simulink model "cst_robotarm"  (R2023b)
settings: Solver=ode23t  StartTime=0.0  StopTime=5  FixedStep=0.0001  MaxStep=0.05  RelTol=1e-3  EnableMultiTasking=on
model workspace (MAT data in the model file):
  DCMotor_J = 0.0946866703633
  DCMotor_K = 0.477771340295
  DCMotor_Kf = 0.921434142151
  DCMotor_L = 0.000316454712175
  DCMotor_R = 4.99938152603
  Ts = 0.1
  dFilt = [1 -0.1202]
  nFilt = [0.4399 0.4399]
undefined symbols (not defined in the file or in its folder): X, Y, Z
libraries: sm_lib x244, fl_lib x75, nesl_utility x28, ee_lib x21, slpidlib x6, SignalEditorBlockLib x1
(part 5 of 7)

== system cst_robotarm/6 DOF Robot Arm/6 DOF Robot Arm Mechanics/Hand/GripAttachmentPlate_1_RIGID ==
  ReferenceFrame : sm_lib/Frames and Transforms/Reference Frame
  Solid : sm_lib/Body Elements/File Solid  ExtGeomFileName=GripAttachmentPlate_Default_sldprt.STL  UnitType=Custom  ExtGeomFileUnits=mm  StepReaderType=HEX  ExportConvexHullGeometry=off  InertiaType=Custom  Mass=0.011413528336954156  MassUnits=kg  CenterOfMass=[0 0 1.5]  CenterOfMassUnits=mm  MomentsOfInertia=[0.70625654823604433 4.0114808704620435 4.7006171261926557]  MomentsOfInertiaUnits=kg*mm^2  ProductsOfInertia=[0 0 0]  ProductsOfInertiaUnits=kg*mm^2  BasedOnType=Density  Density=1000  DensityUnits=kg/(m^3)  DoExposeReferenceFrame=on  SerializedFrames=<Frames/>  GraphicType=FromGeometry  MarkerShape=Sphere  MarkerSize=10  MarkerSizeUnits=m  GraphicVisPropType=SimpleVisualProperties  GraphicDiffuseColor=[1.0 0.8 0.6]  GraphicSpecularColor=[0.5 0.5 0.5 1.0]  GraphicAmbientColor=[0.15 0.15 0.15 1.0]  GraphicEmissiveColor=[0.0 0.0 0.0 1.0]  GraphicShininess=75  GraphicOpacity=1
  F : PMIOPort  Side=Left
  connections:
  Solid/RConn1 -- ReferenceFrame/RConn1 -- F/RConn1

== system cst_robotarm/6 DOF Robot Arm/6 DOF Robot Arm Mechanics/Hand/ServoTJD2_1_RIGID ==
  ReferenceFrame : sm_lib/Frames and Transforms/Reference Frame
  Transform : sm_lib/Frames and Transforms/Rigid Transform  TranslationMethod=None  TranslationStandardOffset=0  TranslationStandardOffsetUnits=m  TranslationStandardAxis=+Z  TranslationCartesianOffset=[0 0 0]  TranslationCartesianOffsetUnits=m  TranslationROffset=0  TranslationROffsetUnits=m  TranslationZOffset=0  TranslationZOffsetUnits=m  TranslationThetaOffset=0  TranslationThetaOffsetUnits=deg  RotationMethod=None  RotationAngleUnits=deg  RotationStandardAxis=+Z  RotationAngle=0.0  RotationArbitraryAxis=[0 0 1]  FollAlignAxisA=+X  BaseAlignAxisA=+Y  FollAlignAxisB=+Y  BaseAlignAxisB=+Z  RotationSequenceAxes=FollowerAxes  RotationSequence=XYX  RotationSequenceAngles=[0 0 0]  RotationSequenceAnglesUnits=deg  RotationMatrix=[1 0 0; 0 1 0; 0 0 1]  Quaternion=[1 0 0 0]
  Transform1 : sm_lib/Frames and Transforms/Rigid Transform  TranslationMethod=Cartesian  TranslationStandardOffset=0  TranslationStandardOffsetUnits=mm  TranslationStandardAxis=+Z  TranslationCartesianOffset=[19.3675 9.8424999999999763 -1.1906249999999998]  TranslationCartesianOffsetUnits=mm  TranslationROffset=0  TranslationROffsetUnits=m  TranslationZOffset=0  TranslationZOffsetUnits=m  TranslationThetaOffset=0  TranslationThetaOffsetUnits=deg  RotationMethod=ArbitraryAxis  RotationAngleUnits=rad  RotationStandardAxis=+Z  RotationAngle=3.1415926535897931  RotationArbitraryAxis=[5.872382563893875e-17 -0.70710678118654746 -0.70710678118654757]  FollAlignAxisA=+X  BaseAlignAxisA=+Y  FollAlignAxisB=+Y  BaseAlignAxisB=+Z  RotationSequenceAxes=FollowerAxes  RotationSequence=XYX  RotationSequenceAngles=[0 0 0]  RotationSequenceAnglesUnits=deg  RotationMatrix=[1 0 0; 0 1 0; 0 0 1]  Quaternion=[1 0 0 0]
  Transform2 : sm_lib/Frames and Transforms/Rigid Transform  TranslationMethod=Cartesian  TranslationStandardOffset=0  TranslationStandardOffsetUnits=mm  TranslationStandardAxis=+Z  TranslationCartesianOffset=[19.367499999999982 9.8424999999999763 -23.8125]  TranslationCartesianOffsetUnits=mm  TranslationROffset=0  TranslationROffsetUnits=m  TranslationZOffset=0  TranslationZOffsetUnits=m  TranslationThetaOffset=0  TranslationThetaOffsetUnits=deg  RotationMethod=ArbitraryAxis  RotationAngleUnits=rad  RotationStandardAxis=+Z  RotationAngle=1.5707963267948968  RotationArbitraryAxis=[1 0 0]  FollAlignAxisA=+X  BaseAlignAxisA=+Y  FollAlignAxisB=+Y  BaseAlignAxisB=+Z  RotationSequenceAxes=FollowerAxes  RotationSequence=XYX  RotationSequenceAngles=[0 0 0]  RotationSequenceAnglesUnits=deg  RotationMatrix=[1 0 0; 0 1 0; 0 0 1]  Quaternion=[1 0 0 0]
  Transform3 : sm_lib/Frames and Transforms/Rigid Transform  TranslationMethod=Cartesian  TranslationStandardOffset=0  TranslationStandardOffsetUnits=mm  TranslationStandardAxis=+Z  TranslationCartesianOffset=[-8.9620000000000051 21.842499999999987 -9.8425000000000029]  TranslationCartesianOffsetUnits=mm  TranslationROffset=0  TranslationROffsetUnits=m  TranslationZOffset=0  TranslationZOffsetUnits=m  TranslationThetaOffset=0  TranslationThetaOffsetUnits=deg  RotationMethod=ArbitraryAxis  RotationAngleUnits=rad  RotationStandardAxis=+Z  RotationAngle=3.1415926535897931  RotationArbitraryAxis=[0.70710678118654746 -2.1920991699290503e-17 0.70710678118654757]  FollAlignAxisA=+X  BaseAlignAxisA=+Y  FollAlignAxisB=+Y  BaseAlignAxisB=+Z  RotationSequenceAxes=FollowerAxes  RotationSequence=XYX  RotationSequenceAngles=[0 0 0]  RotationSequenceAnglesUnits=deg  RotationMatrix=[1 0 0; 0 1 0; 0 0 1]  Quaternion=[1 0 0 0]
  bottom_cover_1_RIGID : Subsystem
  servo_Case_1_RIGID : Subsystem
  servo_cover_2_RIGID : Subsystem
  F : PMIOPort  Side=Right
  connections:
  Transform/RConn1 -- servo_cover_2_RIGID/LConn1
  Transform1/RConn1 -- servo_Case_1_RIGID/LConn1
  Transform2/RConn1 -- bottom_cover_1_RIGID/LConn1
  ReferenceFrame/RConn1 -- Transform/LConn1 -- Transform3/RConn1 -- Transform2/LConn1 -- Transform1/LConn1
  Transform3/LConn1 -- F/RConn1

== system cst_robotarm/6 DOF Robot Arm/6 DOF Robot Arm Mechanics/Hand/gat2_1_RIGID ==
  ReferenceFrame : sm_lib/Frames and Transforms/Reference Frame
  Solid : sm_lib/Body Elements/File Solid  ExtGeomFileName=gat2_Default_sldprt.STL  UnitType=Custom  ExtGeomFileUnits=mm  StepReaderType=HEX  ExportConvexHullGeometry=off  InertiaType=Custom  Mass=0.00050610242376002699  MassUnits=kg  CenterOfMass=[0 0 0]  CenterOfMassUnits=mm  MomentsOfInertia=[0.0015997718916707939 0.027019343024713809 0.028429326507474591]  MomentsOfInertiaUnits=kg*mm^2  ProductsOfInertia=[0 0 0]  ProductsOfInertiaUnits=kg*mm^2  BasedOnType=Density  Density=1000  DensityUnits=kg/(m^3)  DoExposeReferenceFrame=on  SerializedFrames=<Frames/>  GraphicType=FromGeometry  MarkerShape=Sphere  MarkerSize=10  MarkerSizeUnits=m  GraphicVisPropType=SimpleVisualProperties  GraphicDiffuseColor=[1.0 0.8 0.6]  GraphicSpecularColor=[0.5 0.5 0.5 1.0]  GraphicAmbientColor=[0.15 0.15 0.15 1.0]  GraphicEmissiveColor=[0.0 0.0 0.0 1.0]  GraphicShininess=75  GraphicOpacity=1
  F : PMIOPort  Side=Left
  connections:
  Solid/RConn1 -- ReferenceFrame/RConn1 -- F/RConn1

== system cst_robotarm/6 DOF Robot Arm/6 DOF Robot Arm Mechanics/Hand/gat2_2_RIGID ==
  ReferenceFrame : sm_lib/Frames and Transforms/Reference Frame
  Solid : sm_lib/Body Elements/File Solid  ExtGeomFileName=gat2_Default_sldprt.STL  UnitType=Custom  ExtGeomFileUnits=mm  StepReaderType=HEX  ExportConvexHullGeometry=off  InertiaType=Custom  Mass=0.00050610242376002699  MassUnits=kg  CenterOfMass=[0 0 0]  CenterOfMassUnits=mm  MomentsOfInertia=[0.0015997718916707939 0.027019343024713809 0.028429326507474591]  MomentsOfInertiaUnits=kg*mm^2  ProductsOfInertia=[0 0 0]  ProductsOfInertiaUnits=kg*mm^2  BasedOnType=Density  Density=1000  DensityUnits=kg/(m^3)  DoExposeReferenceFrame=on  SerializedFrames=<Frames/>  GraphicType=FromGeometry  MarkerShape=Sphere  MarkerSize=10  MarkerSizeUnits=m  GraphicVisPropType=SimpleVisualProperties  GraphicDiffuseColor=[1.0 0.8 0.6]  GraphicSpecularColor=[0.5 0.5 0.5 1.0]  GraphicAmbientColor=[0.15 0.15 0.15 1.0]  GraphicEmissiveColor=[0.0 0.0 0.0 1.0]  GraphicShininess=75  GraphicOpacity=1
  F : PMIOPort  Side=Left
  connections:
  Solid/RConn1 -- ReferenceFrame/RConn1 -- F/RConn1

== system cst_robotarm/6 DOF Robot Arm/6 DOF Robot Arm Mechanics/Hand/gat3_1_RIGID ==
  ReferenceFrame : sm_lib/Frames and Transforms/Reference Frame
  Solid : sm_lib/Body Elements/File Solid  ExtGeomFileName=gat3_Default_sldprt.STL  UnitType=Custom  ExtGeomFileUnits=mm  StepReaderType=HEX  ExportConvexHullGeometry=off  InertiaType=Custom  Mass=0.013404466225302725  MassUnits=kg  CenterOfMass=[2.3381498585899534 12.0054171558366 0]  CenterOfMassUnits=mm  MomentsOfInertia=[5.9325752245289687 5.0094665513353727 1.34350330449193]  MomentsOfInertiaUnits=kg*mm^2  ProductsOfInertia=[0 0 0.00016978260661059655]  ProductsOfInertiaUnits=kg*mm^2  BasedOnType=Density  Density=1000  DensityUnits=kg/(m^3)  DoExposeReferenceFrame=on  SerializedFrames=<Frames/>  GraphicType=FromGeometry  MarkerShape=Sphere  MarkerSize=10  MarkerSizeUnits=m  GraphicVisPropType=SimpleVisualProperties  GraphicDiffuseColor=[1.0 0.8 0.6]  GraphicSpecularColor=[0.5 0.5 0.5 1.0]  GraphicAmbientColor=[0.15 0.15 0.15 1.0]  GraphicEmissiveColor=[0.0 0.0 0.0 1.0]  GraphicShininess=75  GraphicOpacity=1
  F : PMIOPort  Side=Left
  connections:
  Solid/RConn1 -- ReferenceFrame/RConn1 -- F/RConn1

== system cst_robotarm/6 DOF Robot Arm/6 DOF Robot Arm Mechanics/Hand/lpags_02_1_RIGID ==
  ReferenceFrame : sm_lib/Frames and Transforms/Reference Frame
  SMLINK_HandGearXform : sm_lib/Frames and Transforms/Rigid Transform  TranslationMethod=None  TranslationStandardOffset=0  TranslationStandardOffsetUnits=m  TranslationStandardAxis=+Z  TranslationCartesianOffset=[0 0 0]  TranslationCartesianOffsetUnits=m  TranslationROffset=0  TranslationROffsetUnits=m  TranslationZOffset=0  TranslationZOffsetUnits=m  TranslationThetaOffset=0  TranslationThetaOffsetUnits=deg  RotationMethod=None  RotationAngleUnits=deg  RotationStandardAxis=+Z  RotationAngle=0.0  RotationArbitraryAxis=[0 0 1]  FollAlignAxisA=+X  BaseAlignAxisA=+Y  FollAlignAxisB=+Y  BaseAlignAxisB=+Z  RotationSequenceAxes=FollowerAxes  RotationSequence=XYX  RotationSequenceAngles=[0 0 0]  RotationSequenceAnglesUnits=deg  RotationMatrix=[1 0 0; 0 1 0; 0 0 1]  Quaternion=[1 0 0 0]
  Solid : sm_lib/Body Elements/File Solid  ExtGeomFileName=lpags-02_Default_sldprt.STL  UnitType=Custom  ExtGeomFileUnits=mm  StepReaderType=HEX  ExportConvexHullGeometry=off  InertiaType=Custom  Mass=0.0030318967834451023  MassUnits=kg  CenterOfMass=[0 0.57150000000000001 -0.00019934083817513303]  CenterOfMassUnits=mm  MomentsOfInertia=[0.31419992840808614 0.62773233420718355 0.31419225543277651]  MomentsOfInertiaUnits=kg*mm^2  ProductsOfInertia=[0 0 8.0061496389648527e-09]  ProductsOfInertiaUnits=kg*mm^2  BasedOnType=Density  Density=1000  DensityUnits=kg/(m^3)  DoExposeReferenceFrame=on  SerializedFrames=<Frames/>  GraphicType=FromGeometry  MarkerShape=Sphere  MarkerSize=10  MarkerSizeUnits=m  GraphicVisPropType=SimpleVisualProperties  GraphicDiffuseColor=[1.0 1.0 1.0]  GraphicSpecularColor=[0.5 0.5 0.5 1.0]  GraphicAmbientColor=[0.15 0.15 0.15 1.0]  GraphicEmissiveColor=[0.0 0.0 0.0 1.0]  GraphicShininess=75  GraphicOpacity=1
  F : PMIOPort  Side=Left
  SMLINK_HandGear : PMIOPort  Port=2  Side=Right
  connections:
  SMLINK_HandGearXform/LConn1 -- ReferenceFrame/RConn1 -- F/RConn1 -- Solid/RConn1
  SMLINK_HandGearXform/RConn1 -- SMLINK_HandGear/RConn1

== system cst_robotarm/6 DOF Robot Arm/6 DOF Robot Arm Mechanics/Turntable/ServoTJD_1_RIGID ==
  ReferenceFrame : sm_lib/Frames and Transforms/Reference Frame
  ServoHornPlastic_1_RIGID : Subsystem
  Transform : sm_lib/Frames and Transforms/Rigid Transform  TranslationMethod=None  TranslationStandardOffset=0  TranslationStandardOffsetUnits=m  TranslationStandardAxis=+Z  TranslationCartesianOffset=[0 0 0]  TranslationCartesianOffsetUnits=m  TranslationROffset=0  TranslationROffsetUnits=m  TranslationZOffset=0  TranslationZOffsetUnits=m  TranslationThetaOffset=0  TranslationThetaOffsetUnits=deg  RotationMethod=None  RotationAngleUnits=deg  RotationStandardAxis=+Z  RotationAngle=0.0  RotationArbitraryAxis=[0 0 1]  FollAlignAxisA=+X  BaseAlignAxisA=+Y  FollAlignAxisB=+Y  BaseAlignAxisB=+Z  RotationSequenceAxes=FollowerAxes  RotationSequence=XYX  RotationSequenceAngles=[0 0 0]  RotationSequenceAnglesUnits=deg  RotationMatrix=[1 0 0; 0 1 0; 0 0 1]  Quaternion=[1 0 0 0]
  Transform1 : sm_lib/Frames and Transforms/Rigid Transform  TranslationMethod=Cartesian  TranslationStandardOffset=0  TranslationStandardOffsetUnits=mm  TranslationStandardAxis=+Z  TranslationCartesianOffset=[19.367500000000003 9.8425000000000047 -1.1906250000000007]  TranslationCartesianOffsetUnits=mm  TranslationROffset=0  TranslationROffsetUnits=m  TranslationZOffset=0  TranslationZOffsetUnits=m  TranslationThetaOffset=0  TranslationThetaOffsetUnits=deg  RotationMethod=ArbitraryAxis  RotationAngleUnits=rad  RotationStandardAxis=+Z  RotationAngle=3.1415926535897931  RotationArbitraryAxis=[5.8878467200641572e-17 -0.70710678118654746 -0.70710678118654757]  FollAlignAxisA=+X  BaseAlignAxisA=+Y  FollAlignAxisB=+Y  BaseAlignAxisB=+Z  RotationSequenceAxes=FollowerAxes  RotationSequence=XYX  RotationSequenceAngles=[0 0 0]  RotationSequenceAnglesUnits=deg  RotationMatrix=[1 0 0; 0 1 0; 0 0 1]  Quaternion=[1 0 0 0]
  Transform2 : sm_lib/Frames and Transforms/Rigid Transform  TranslationMethod=Cartesian  TranslationStandardOffset=0  TranslationStandardOffsetUnits=mm  TranslationStandardAxis=+Z  TranslationCartesianOffset=[19.367499999999989 9.8425000000000047 -23.812500000000007]  TranslationCartesianOffsetUnits=mm  TranslationROffset=0  TranslationROffsetUnits=m  TranslationZOffset=0  TranslationZOffsetUnits=m  TranslationThetaOffset=0  TranslationThetaOffsetUnits=deg  RotationMethod=ArbitraryAxis  RotationAngleUnits=rad  RotationStandardAxis=+Z  RotationAngle=1.5707963267948968  RotationArbitraryAxis=[1 0 0]  FollAlignAxisA=+X  BaseAlignAxisA=+Y  FollAlignAxisB=+Y  BaseAlignAxisB=+Z  RotationSequenceAxes=FollowerAxes  RotationSequence=XYX  RotationSequenceAngles=[0 0 0]  RotationSequenceAnglesUnits=deg  RotationMatrix=[1 0 0; 0 1 0; 0 0 1]  Quaternion=[1 0 0 0]
  Transform3 : sm_lib/Frames and Transforms/Rigid Transform  TranslationMethod=Cartesian  TranslationStandardOffset=0  TranslationStandardOffsetUnits=mm  TranslationStandardAxis=+Z  TranslationCartesianOffset=[9.8425000000000029 9.8425000000000047 17.962]  TranslationCartesianOffsetUnits=mm  TranslationROffset=0  TranslationROffsetUnits=m  TranslationZOffset=0  TranslationZOffsetUnits=m  TranslationThetaOffset=0  TranslationThetaOffsetUnits=deg  RotationMethod=ArbitraryAxis  RotationAngleUnits=rad  RotationStandardAxis=+Z  RotationAngle=1.5707963267948968  RotationArbitraryAxis=[1 0 0]  FollAlignAxisA=+X  BaseAlignAxisA=+Y  FollAlignAxisB=+Y  BaseAlignAxisB=+Z  RotationSequenceAxes=FollowerAxes  RotationSequence=XYX  RotationSequenceAngles=[0 0 0]  RotationSequenceAnglesUnits=deg  RotationMatrix=[1 0 0; 0 1 0; 0 0 1]  Quaternion=[1 0 0 0]
  Transform4 : sm_lib/Frames and Transforms/Rigid Transform  TranslationMethod=Cartesian  TranslationStandardOffset=0  TranslationStandardOffsetUnits=mm  TranslationStandardAxis=+Z  TranslationCartesianOffset=[30.38750000000001 -48.386999999999396 8.9609000000000876]  TranslationCartesianOffsetUnits=mm  TranslationROffset=0  TranslationROffsetUnits=m  TranslationZOffset=0  TranslationZOffsetUnits=m  TranslationThetaOffset=0  TranslationThetaOffsetUnits=deg  RotationMethod=ArbitraryAxis  RotationAngleUnits=rad  RotationStandardAxis=+Z  RotationAngle=2.0943951023931939  RotationArbitraryAxis=[-0.5773502691896254 -0.57735026918962518 -0.57735026918962684]  FollAlignAxisA=+X  BaseAlignAxisA=+Y  FollAlignAxisB=+Y  BaseAlignAxisB=+Z  RotationSequenceAxes=FollowerAxes  RotationSequence=XYX  RotationSequenceAngles=[0 0 0]  RotationSequenceAnglesUnits=deg  RotationMatrix=[1 0 0; 0 1 0; 0 0 1]  Quaternion=[1 0 0 0]
  bottom_cover_1_RIGID : Subsystem
  servo_Case_1_RIGID : Subsystem
  servo_cover_2_RIGID : Subsystem
  F : PMIOPort  Side=Right
  connections:
  Transform/RConn1 -- servo_cover_2_RIGID/LConn1
  Transform1/RConn1 -- servo_Case_1_RIGID/LConn1
  Transform2/RConn1 -- bottom_cover_1_RIGID/LConn1
  ServoHornPlastic_1_RIGID/LConn1 -- Transform3/RConn1
  ReferenceFrame/RConn1 -- Transform/LConn1 -- Transform1/LConn1 -- Transform4/RConn1 -- Transform3/LConn1 -- Transform2/LConn1
  Transform4/LConn1 -- F/RConn1

== system cst_robotarm/6 DOF Robot Arm/6 DOF Robot Arm Mechanics/Turntable/ServoTJD_2_RIGID ==
  ReferenceFrame : sm_lib/Frames and Transforms/Reference Frame
  ServoHornPlastic_1_RIGID : Subsystem
  Transform : sm_lib/Frames and Transforms/Rigid Transform  TranslationMethod=None  TranslationStandardOffset=0  TranslationStandardOffsetUnits=m  TranslationStandardAxis=+Z  TranslationCartesianOffset=[0 0 0]  TranslationCartesianOffsetUnits=m  TranslationROffset=0  TranslationROffsetUnits=m  TranslationZOffset=0  TranslationZOffsetUnits=m  TranslationThetaOffset=0  TranslationThetaOffsetUnits=deg  RotationMethod=None  RotationAngleUnits=deg  RotationStandardAxis=+Z  RotationAngle=0.0  RotationArbitraryAxis=[0 0 1]  FollAlignAxisA=+X  BaseAlignAxisA=+Y  FollAlignAxisB=+Y  BaseAlignAxisB=+Z  RotationSequenceAxes=FollowerAxes  RotationSequence=XYX  RotationSequenceAngles=[0 0 0]  RotationSequenceAnglesUnits=deg  RotationMatrix=[1 0 0; 0 1 0; 0 0 1]  Quaternion=[1 0 0 0]
  Transform1 : sm_lib/Frames and Transforms/Rigid Transform  TranslationMethod=Cartesian  TranslationStandardOffset=0  TranslationStandardOffsetUnits=mm  TranslationStandardAxis=+Z  TranslationCartesianOffset=[19.36750000000001 9.8424999999999905 -1.1906250000000007]  TranslationCartesianOffsetUnits=mm  TranslationROffset=0  TranslationROffsetUnits=m  TranslationZOffset=0  TranslationZOffsetUnits=m  TranslationThetaOffset=0  TranslationThetaOffsetUnits=deg  RotationMethod=ArbitraryAxis  RotationAngleUnits=rad  RotationStandardAxis=+Z  RotationAngle=3.1415926535897931  RotationArbitraryAxis=[4.5974986977188573e-17 -0.70710678118654746 -0.70710678118654757]  FollAlignAxisA=+X  BaseAlignAxisA=+Y  FollAlignAxisB=+Y  BaseAlignAxisB=+Z  RotationSequenceAxes=FollowerAxes  RotationSequence=XYX  RotationSequenceAngles=[0 0 0]  RotationSequenceAnglesUnits=deg  RotationMatrix=[1 0 0; 0 1 0; 0 0 1]  Quaternion=[1 0 0 0]
  Transform2 : sm_lib/Frames and Transforms/Rigid Transform  TranslationMethod=Cartesian  TranslationStandardOffset=0  TranslationStandardOffsetUnits=mm  TranslationStandardAxis=+Z  TranslationCartesianOffset=[19.367499999999993 9.8425000000000047 -23.8125]  TranslationCartesianOffsetUnits=mm  TranslationROffset=0  TranslationROffsetUnits=m  TranslationZOffset=0  TranslationZOffsetUnits=m  TranslationThetaOffset=0  TranslationThetaOffsetUnits=deg  RotationMethod=ArbitraryAxis  RotationAngleUnits=rad  RotationStandardAxis=+Z  RotationAngle=1.5707963267948968  RotationArbitraryAxis=[1 0 0]  FollAlignAxisA=+X  BaseAlignAxisA=+Y  FollAlignAxisB=+Y  BaseAlignAxisB=+Z  RotationSequenceAxes=FollowerAxes  RotationSequence=XYX  RotationSequenceAngles=[0 0 0]  RotationSequenceAnglesUnits=deg  RotationMatrix=[1 0 0; 0 1 0; 0 0 1]  Quaternion=[1 0 0 0]
  Transform3 : sm_lib/Frames and Transforms/Rigid Transform  TranslationMethod=Cartesian  TranslationStandardOffset=0  TranslationStandardOffsetUnits=mm  TranslationStandardAxis=+Z  TranslationCartesianOffset=[9.8425000000000047 9.8424999999999905 17.962000000000007]  TranslationCartesianOffsetUnits=mm  TranslationROffset=0  TranslationROffsetUnits=m  TranslationZOffset=0  TranslationZOffsetUnits=m  TranslationThetaOffset=0  TranslationThetaOffsetUnits=deg  RotationMethod=ArbitraryAxis  RotationAngleUnits=rad  RotationStandardAxis=+Z  RotationAngle=1.5707963267948968  RotationArbitraryAxis=[1 0 0]  FollAlignAxisA=+X  BaseAlignAxisA=+Y  FollAlignAxisB=+Y  BaseAlignAxisB=+Z  RotationSequenceAxes=FollowerAxes  RotationSequence=XYX  RotationSequenceAngles=[0 0 0]  RotationSequenceAnglesUnits=deg  RotationMatrix=[1 0 0; 0 1 0; 0 0 1]  Quaternion=[1 0 0 0]
  Transform4 : sm_lib/Frames and Transforms/Rigid Transform  TranslationMethod=Cartesian  TranslationStandardOffset=0  TranslationStandardOffsetUnits=mm  TranslationStandardAxis=+Z  TranslationCartesianOffset=[30.387499999999971 2.4257000000008517 8.9608999999998762]  TranslationCartesianOffsetUnits=mm  TranslationROffset=0  TranslationROffsetUnits=m  TranslationZOffset=0  TranslationZOffsetUnits=m  TranslationThetaOffset=0  TranslationThetaOffsetUnits=deg  RotationMethod=ArbitraryAxis  RotationAngleUnits=rad  RotationStandardAxis=+Z  RotationAngle=2.0943951023931944  RotationArbitraryAxis=[-0.57735026918962506 -0.57735026918962529 -0.57735026918962684]  FollAlignAxisA=+X  BaseAlignAxisA=+Y  FollAlignAxisB=+Y  BaseAlignAxisB=+Z  RotationSequenceAxes=FollowerAxes  RotationSequence=XYX  RotationSequenceAngles=[0 0 0]  RotationSequenceAnglesUnits=deg  RotationMatrix=[1 0 0; 0 1 0; 0 0 1]  Quaternion=[1 0 0 0]
  bottom_cover_1_RIGID : Subsystem
  servo_Case_1_RIGID : Subsystem
  servo_cover_2_RIGID : Subsystem
  F : PMIOPort  Side=Right
  connections:
  Transform/RConn1 -- servo_cover_2_RIGID/LConn1
  Transform1/RConn1 -- servo_Case_1_RIGID/LConn1
  Transform2/RConn1 -- bottom_cover_1_RIGID/LConn1
  ServoHornPlastic_1_RIGID/LConn1 -- Transform3/RConn1
  Transform/LConn1 -- ReferenceFrame/RConn1 -- Transform4/RConn1 -- Transform3/LConn1 -- Transform2/LConn1 -- Transform1/LConn1
  Transform4/LConn1 -- F/RConn1

== system cst_robotarm/6 DOF Robot Arm/6 DOF Robot Arm Mechanics/Turntable/TurntableBase_1_RIGID ==
  ReferenceFrame : sm_lib/Frames and Transforms/Reference Frame
  Solid : sm_lib/Body Elements/File Solid  ExtGeomFileName=TurntableBase_Default_sldprt.STL  UnitType=Custom  ExtGeomFileUnits=mm  StepReaderType=HEX  ExportConvexHullGeometry=off  InertiaType=Custom  Mass=0.061984090111562314  MassUnits=kg  CenterOfMass=[0 8.3537655787743348e-13 -9.8678648861571805]  CenterOfMassUnits=mm  MomentsOfInertia=[22.766528568089555 51.610594449827772 34.871884065003805]  MomentsOfInertiaUnits=kg*mm^2  ProductsOfInertia=[0 0 0]  ProductsOfInertiaUnits=kg*mm^2  BasedOnType=Density  Density=1000  DensityUnits=kg/(m^3)  DoExposeReferenceFrame=on  SerializedFrames=<Frames/>  GraphicType=FromGeometry  MarkerShape=Sphere  MarkerSize=10  MarkerSizeUnits=m  GraphicVisPropType=SimpleVisualProperties  GraphicDiffuseColor=[0.8 0.8 0.8]  GraphicSpecularColor=[0.5 0.5 0.5 1.0]  GraphicAmbientColor=[0.15 0.15 0.15 1.0]  GraphicEmissiveColor=[0.0 0.0 0.0 1.0]  GraphicShininess=75  GraphicOpacity=1
  F : PMIOPort  Side=Left
  connections:
  Solid/RConn1 -- ReferenceFrame/RConn1 -- F/RConn1

== system cst_robotarm/6 DOF Robot Arm/6 DOF Robot Arm Mechanics/Turntable/TurntablePlate_1_RIGID ==
  ReferenceFrame : sm_lib/Frames and Transforms/Reference Frame
  Solid : sm_lib/Body Elements/File Solid  ExtGeomFileName=TurntablePlate_Default_sldprt.STL  UnitType=Custom  ExtGeomFileUnits=mm  StepReaderType=HEX  ExportConvexHullGeometry=off  InertiaType=Custom  Mass=0.017394579990693507  MassUnits=kg  CenterOfMass=[28.782349121413723 2.6365798461097167 -30.489563019987546]  CenterOfMassUnits=mm  MomentsOfInertia=[6.1456876544929333 11.14133340240272 5.8740116461995679]  MomentsOfInertiaUnits=kg*mm^2  ProductsOfInertia=[-0.010484087253259841 -0.065628305606111978 0.0066466281662198451]  ProductsOfInertiaUnits=kg*mm^2  BasedOnType=Density  Density=1000  DensityUnits=kg/(m^3)  DoExposeReferenceFrame=on  SerializedFrames=<Frames/>  GraphicType=FromGeometry  MarkerShape=Sphere  MarkerSize=10  MarkerSizeUnits=m  GraphicVisPropType=SimpleVisualProperties  GraphicDiffuseColor=[0.8 0.8 0.8]  GraphicSpecularColor=[0.5 0.5 0.5 1.0]  GraphicAmbientColor=[0.15 0.15 0.15 1.0]  GraphicEmissiveColor=[0.0 0.0 0.0 1.0]  GraphicShininess=75  GraphicOpacity=1
  F : PMIOPort  Side=Left
  connections:
  Solid/RConn1 -- ReferenceFrame/RConn1 -- F/RConn1

== system cst_robotarm/6 DOF Robot Arm/6 DOF Robot Arm Mechanics/Wrist/MotorWristAsm_1_RIGID ==
  BB_01_1_RIGID : Subsystem
  ReferenceFrame : sm_lib/Frames and Transforms/Reference Frame
  ServoTJD2_1_RIGID : Subsystem
  Transform : sm_lib/Frames and Transforms/Rigid Transform  TranslationMethod=Cartesian  TranslationStandardOffset=0  TranslationStandardOffsetUnits=mm  TranslationStandardAxis=+Z  TranslationCartesianOffset=[49.387968408803829 0 4.318000000000044]  TranslationCartesianOffsetUnits=mm  TranslationROffset=0  TranslationROffsetUnits=m  TranslationZOffset=0  TranslationZOffsetUnits=m  TranslationThetaOffset=0  TranslationThetaOffsetUnits=deg  RotationMethod=ArbitraryAxis  RotationAngleUnits=rad  RotationStandardAxis=+Z  RotationAngle=2.0943951023931953  RotationArbitraryAxis=[0.57735026918962573 0.57735026918962573 0.57735026918962584]  FollAlignAxisA=+X  BaseAlignAxisA=+Y  FollAlignAxisB=+Y  BaseAlignAxisB=+Z  RotationSequenceAxes=FollowerAxes  RotationSequence=XYX  RotationSequenceAngles=[0 0 0]  RotationSequenceAnglesUnits=deg  RotationMatrix=[1 0 0; 0 1 0; 0 0 1]  Quaternion=[1 0 0 0]
  Transform1 : sm_lib/Frames and Transforms/Rigid Transform  TranslationMethod=Cartesian  TranslationStandardOffset=0  TranslationStandardOffsetUnits=mm  TranslationStandardAxis=+Z  TranslationCartesianOffset=[8.9130684088038343 49.720500000000008 5.8420000000000138]  TranslationCartesianOffsetUnits=mm  TranslationROffset=0  TranslationROffsetUnits=m  TranslationZOffset=0  TranslationZOffsetUnits=m  TranslationThetaOffset=0  TranslationThetaOffsetUnits=deg  RotationMethod=None  RotationAngleUnits=deg  RotationStandardAxis=+Z  RotationAngle=0.0  RotationArbitraryAxis=[0 0 1]  FollAlignAxisA=+X  BaseAlignAxisA=+Y  FollAlignAxisB=+Y  BaseAlignAxisB=+Z  RotationSequenceAxes=FollowerAxes  RotationSequence=XYX  RotationSequenceAngles=[0 0 0]  RotationSequenceAnglesUnits=deg  RotationMatrix=[1 0 0; 0 1 0; 0 0 1]  Quaternion=[1 0 0 0]
  Transform2 : sm_lib/Frames and Transforms/Rigid Transform  TranslationMethod=Cartesian  TranslationStandardOffset=0  TranslationStandardOffsetUnits=mm  TranslationStandardAxis=+Z  TranslationCartesianOffset=[-49.720500000000015 4.318000000000044 8.913068408803829]  TranslationCartesianOffsetUnits=mm  TranslationROffset=0  TranslationROffsetUnits=m  TranslationZOffset=0  TranslationZOffsetUnits=m  TranslationThetaOffset=0  TranslationThetaOffsetUnits=deg  RotationMethod=ArbitraryAxis  RotationAngleUnits=rad  RotationStandardAxis=+Z  RotationAngle=2.0943951023931953  RotationArbitraryAxis=[0.57735026918962584 0.57735026918962573 -0.57735026918962573]  FollAlignAxisA=+X  BaseAlignAxisA=+Y  FollAlignAxisB=+Y  BaseAlignAxisB=+Z  RotationSequenceAxes=FollowerAxes  RotationSequence=XYX  RotationSequenceAngles=[0 0 0]  RotationSequenceAnglesUnits=deg  RotationMatrix=[1 0 0; 0 1 0; 0 0 1]  Quaternion=[1 0 0 0]
  asb_14_2_RIGID : Subsystem
  F : PMIOPort  Side=Right
  connections:
  Transform/RConn1 -- asb_14_2_RIGID/LConn1
  BB_01_1_RIGID/LConn1 -- Transform1/RConn1
  ReferenceFrame/RConn1 -- ServoTJD2_1_RIGID/LConn1 -- Transform2/RConn1 -- Transform1/LConn1 -- Transform/LConn1
  Transform2/LConn1 -- F/RConn1

== system cst_robotarm/6 DOF Robot Arm/6 DOF Robot Arm Mechanics/Wrist/asb_09_1_RIGID ==
  ReferenceFrame : sm_lib/Frames and Transforms/Reference Frame
  Solid : sm_lib/Body Elements/File Solid  ExtGeomFileName=asb-09_Default_sldprt.STL  UnitType=Custom  ExtGeomFileUnits=mm  StepReaderType=HEX  ExportConvexHullGeometry=off  InertiaType=Custom  Mass=0.012849741350911532  MassUnits=kg  CenterOfMass=[0 11.553213185970444 0]  CenterOfMassUnits=mm  MomentsOfInertia=[2.609817980818478 6.7181730593401783 8.0141886683045769]  MomentsOfInertiaUnits=kg*mm^2  ProductsOfInertia=[0 0 0]  ProductsOfInertiaUnits=kg*mm^2  BasedOnType=Density  Density=1000  DensityUnits=kg/(m^3)  DoExposeReferenceFrame=on  SerializedFrames=<Frames/>  GraphicType=FromGeometry  MarkerShape=Sphere  MarkerSize=10  MarkerSizeUnits=m  GraphicVisPropType=SimpleVisualProperties  GraphicDiffuseColor=[0.8 1.0 0.6]  GraphicSpecularColor=[0.5 0.5 0.5 1.0]  GraphicAmbientColor=[0.15 0.15 0.15 1.0]  GraphicEmissiveColor=[0.0 0.0 0.0 1.0]  GraphicShininess=75  GraphicOpacity=1
  F : PMIOPort  Side=Left
  connections:
  Solid/RConn1 -- ReferenceFrame/RConn1 -- F/RConn1

== system cst_robotarm/6 DOF Robot Arm/DC Motors/Bicep Motor1/Power Amplifier ==
  Duty : Inport
  REV : Inport  Port=2
  BRK : Inport  Port=3
  Controlled PWM Voltage : ee_lib/Integrated Circuits/Controlled PWM Voltage  F=400 Hz  TD=0 s  pulse_width_offset=0 s  pulse_min=0 s  pwm_or_av=2  event_type=1  sample_time=1e-6 s  Vmin=0 V  Vmax=5 V  Vm=5 V  u_min=0  u_max=1
  Electrical Reference1 : fl_lib/Electrical/Electrical Elements/Electrical Reference
  H-Bridge : ee_lib/Semiconductors & Converters/Converters/H-Bridge  supply_ports=ee.enum.supply_ports.hidesupply  pwm_or_av=2  regenerative_braking_mode=2  discontinuous=0  freewheeling_mode=1  Rload=10 Ohm  Lload=1e-5 H  F=10 kHz  Venable=2.5 V  Vmax=5 V  Vreverse=2.5 V  Vbrake=2.5 V  Vm=12 V  Ron=0.1 Ohm  Don=0.05 Ohm  Goff=1e-6 S  Tmeas=298.15 K  Ron2=0.1 Ohm  Don2=0.05 Ohm  Tmeas2=398.15 K  thermal_mass=100 J/K  initial_temperature=298.15 K
  SL2Vbrk : Subsystem
  SL2Vduty : Subsystem
  SL2Vrev : Subsystem
  V + : PMIOPort  Tag=PMCPort  Side=Right
  V -- : PMIOPort  Tag=PMCPort  Port=2  Side=Right
  wires:
  BRK/1 -> SL2Vbrk/1(Signal)
  REV/1 -> SL2Vrev/1(Signal)
  Duty/1 -> SL2Vduty/1(Signal)
  connections:
  SL2Vbrk/RConn1 -- H-Bridge/LConn4
  H-Bridge/LConn1 -- Controlled PWM Voltage/RConn1
  SL2Vduty/RConn1 -- Controlled PWM Voltage/LConn1
  H-Bridge/RConn1 -- V +/RConn1
  SL2Vrev/RConn1 -- H-Bridge/LConn3
  H-Bridge/LConn2 -- Controlled PWM Voltage/LConn2 -- Electrical Reference1/LConn1 -- V --/RConn1 -- H-Bridge/RConn2 -- Controlled PWM Voltage/RConn2

== system cst_robotarm/6 DOF Robot Arm/DC Motors/Bicep Motor2/Power Amplifier ==
  Duty : Inport
  REV : Inport  Port=2
  BRK : Inport  Port=3
  Controlled PWM Voltage : ee_lib/Integrated Circuits/Controlled PWM Voltage  F=400 Hz  TD=0 s  pulse_width_offset=0 s  pulse_min=0 s  pwm_or_av=2  event_type=1  sample_time=1e-6 s  Vmin=0 V  Vmax=5 V  Vm=5 V  u_min=0  u_max=1
  Electrical Reference1 : fl_lib/Electrical/Electrical Elements/Electrical Reference
  H-Bridge : ee_lib/Semiconductors & Converters/Converters/H-Bridge  supply_ports=ee.enum.supply_ports.hidesupply  pwm_or_av=2  regenerative_braking_mode=2  discontinuous=0  freewheeling_mode=1  Rload=10 Ohm  Lload=1e-5 H  F=10 kHz  Venable=2.5 V  Vmax=5 V  Vreverse=2.5 V  Vbrake=2.5 V  Vm=12 V  Ron=0.1 Ohm  Don=0.05 Ohm  Goff=1e-6 S  Tmeas=298.15 K  Ron2=0.1 Ohm  Don2=0.05 Ohm  Tmeas2=398.15 K  thermal_mass=100 J/K  initial_temperature=298.15 K
  SL2Vbrk : Subsystem
  SL2Vduty : Subsystem
  SL2Vrev : Subsystem
  V + : PMIOPort  Tag=PMCPort  Side=Right
  V -- : PMIOPort  Tag=PMCPort  Port=2  Side=Right
  wires:
  Duty/1 -> SL2Vduty/1(Signal)
  REV/1 -> SL2Vrev/1(Signal)
  BRK/1 -> SL2Vbrk/1(Signal)
  connections:
  Controlled PWM Voltage/RConn2 -- H-Bridge/RConn2 -- V --/RConn1 -- Electrical Reference1/LConn1 -- Controlled PWM Voltage/LConn2 -- H-Bridge/LConn2
  SL2Vrev/RConn1 -- H-Bridge/LConn3
  H-Bridge/RConn1 -- V +/RConn1
  SL2Vduty/RConn1 -- Controlled PWM Voltage/LConn1
  H-Bridge/LConn1 -- Controlled PWM Voltage/RConn1
  SL2Vbrk/RConn1 -- H-Bridge/LConn4

== system cst_robotarm/6 DOF Robot Arm/DC Motors/Forearm Motor/Power Amplifier ==
  Duty : Inport
  REV : Inport  Port=2
  BRK : Inport  Port=3
  Controlled PWM Voltage : ee_lib/Integrated Circuits/Controlled PWM Voltage  F=400 Hz  TD=0 s  pulse_width_offset=0 s  pulse_min=0 s  pwm_or_av=2  event_type=1  sample_time=1e-6 s  Vmin=0 V  Vmax=5 V  Vm=5 V  u_min=0  u_max=1
  Electrical Reference1 : fl_lib/Electrical/Electrical Elements/Electrical Reference
  H-Bridge : ee_lib/Semiconductors & Converters/Converters/H-Bridge  supply_ports=ee.enum.supply_ports.hidesupply  pwm_or_av=2  regenerative_braking_mode=2  discontinuous=0  freewheeling_mode=1  Rload=10 Ohm  Lload=1e-5 H  F=10 kHz  Venable=2.5 V  Vmax=5 V  Vreverse=2.5 V  Vbrake=2.5 V  Vm=12 V  Ron=0.1 Ohm  Don=0.05 Ohm  Goff=1e-6 S  Tmeas=298.15 K  Ron2=0.1 Ohm  Don2=0.05 Ohm  Tmeas2=398.15 K  thermal_mass=100 J/K  initial_temperature=298.15 K
  SL2Vbrk : Subsystem
  SL2Vduty : Subsystem
  SL2Vrev : Subsystem
  V + : PMIOPort  Tag=PMCPort  Side=Right
  V -- : PMIOPort  Tag=PMCPort  Port=2  Side=Right
  wires:
  Duty/1 -> SL2Vduty/1(Signal)
  REV/1 -> SL2Vrev/1(Signal)
  BRK/1 -> SL2Vbrk/1(Signal)
  connections:
  Controlled PWM Voltage/RConn2 -- H-Bridge/RConn2 -- V --/RConn1 -- Electrical Reference1/LConn1 -- Controlled PWM Voltage/LConn2 -- H-Bridge/LConn2
  SL2Vrev/RConn1 -- H-Bridge/LConn3
  H-Bridge/RConn1 -- V +/RConn1
  SL2Vduty/RConn1 -- Controlled PWM Voltage/LConn1
  H-Bridge/LConn1 -- Controlled PWM Voltage/RConn1
  SL2Vbrk/RConn1 -- H-Bridge/LConn4

== system cst_robotarm/6 DOF Robot Arm/DC Motors/Hand Motor/Power Amplifier ==
  Duty : Inport
  REV : Inport  Port=2
  BRK : Inport  Port=3
  Controlled PWM Voltage : ee_lib/Integrated Circuits/Controlled PWM Voltage  F=400 Hz  TD=0 s  pulse_width_offset=0 s  pulse_min=0 s  pwm_or_av=2  event_type=1  sample_time=1e-6 s  Vmin=0 V  Vmax=5 V  Vm=5 V  u_min=0  u_max=1
  Electrical Reference1 : fl_lib/Electrical/Electrical Elements/Electrical Reference
  H-Bridge : ee_lib/Semiconductors & Converters/Converters/H-Bridge  supply_ports=ee.enum.supply_ports.hidesupply  pwm_or_av=2  regenerative_braking_mode=2  discontinuous=0  freewheeling_mode=1  Rload=10 Ohm  Lload=1e-5 H  F=10 kHz  Venable=2.5 V  Vmax=5 V  Vreverse=2.5 V  Vbrake=2.5 V  Vm=12 V  Ron=0.1 Ohm  Don=0.05 Ohm  Goff=1e-6 S  Tmeas=298.15 K  Ron2=0.1 Ohm  Don2=0.05 Ohm  Tmeas2=398.15 K  thermal_mass=100 J/K  initial_temperature=298.15 K
  SL2Vbrk : Subsystem
  SL2Vduty : Subsystem
  SL2Vrev : Subsystem
  V + : PMIOPort  Tag=PMCPort  Side=Right
  V -- : PMIOPort  Tag=PMCPort  Port=2  Side=Right
  wires:
  Duty/1 -> SL2Vduty/1(Signal)
  REV/1 -> SL2Vrev/1(Signal)
  BRK/1 -> SL2Vbrk/1(Signal)
  connections:
  Controlled PWM Voltage/RConn2 -- H-Bridge/RConn2 -- V --/RConn1 -- Electrical Reference1/LConn1 -- Controlled PWM Voltage/LConn2 -- H-Bridge/LConn2
  SL2Vrev/RConn1 -- H-Bridge/LConn3
  H-Bridge/RConn1 -- V +/RConn1
  SL2Vduty/RConn1 -- Controlled PWM Voltage/LConn1
  H-Bridge/LConn1 -- Controlled PWM Voltage/RConn1
  SL2Vbrk/RConn1 -- H-Bridge/LConn4

== system cst_robotarm/6 DOF Robot Arm/DC Motors/Hand Motor1/Power Amplifier ==
  Duty : Inport
  REV : Inport  Port=2
  BRK : Inport  Port=3
  Controlled PWM Voltage : ee_lib/Integrated Circuits/Controlled PWM Voltage  F=400 Hz  TD=0 s  pulse_width_offset=0 s  pulse_min=0 s  pwm_or_av=2  event_type=1  sample_time=1e-6 s  Vmin=0 V  Vmax=5 V  Vm=5 V  u_min=0  u_max=1
  Electrical Reference1 : fl_lib/Electrical/Electrical Elements/Electrical Reference
  H-Bridge : ee_lib/Semiconductors & Converters/Converters/H-Bridge  supply_ports=ee.enum.supply_ports.hidesupply  pwm_or_av=2  regenerative_braking_mode=2  discontinuous=0  freewheeling_mode=1  Rload=10 Ohm  Lload=1e-5 H  F=10 kHz  Venable=2.5 V  Vmax=5 V  Vreverse=2.5 V  Vbrake=2.5 V  Vm=12 V  Ron=0.1 Ohm  Don=0.05 Ohm  Goff=1e-6 S  Tmeas=298.15 K  Ron2=0.1 Ohm  Don2=0.05 Ohm  Tmeas2=398.15 K  thermal_mass=100 J/K  initial_temperature=298.15 K
  SL2Vbrk : Subsystem
  SL2Vduty : Subsystem
  SL2Vrev : Subsystem
  V + : PMIOPort  Tag=PMCPort  Side=Right
  V -- : PMIOPort  Tag=PMCPort  Port=2  Side=Right
  wires:
  BRK/1 -> SL2Vbrk/1(Signal)
  REV/1 -> SL2Vrev/1(Signal)
  Duty/1 -> SL2Vduty/1(Signal)
  connections:
  SL2Vbrk/RConn1 -- H-Bridge/LConn4
  H-Bridge/LConn1 -- Controlled PWM Voltage/RConn1
  SL2Vduty/RConn1 -- Controlled PWM Voltage/LConn1
  H-Bridge/RConn1 -- V +/RConn1
  SL2Vrev/RConn1 -- H-Bridge/LConn3
  H-Bridge/LConn2 -- Controlled PWM Voltage/LConn2 -- Electrical Reference1/LConn1 -- V --/RConn1 -- H-Bridge/RConn2 -- Controlled PWM Voltage/RConn2

== system cst_robotarm/6 DOF Robot Arm/DC Motors/Turntable Motor/Power Amplifier ==
  Duty : Inport
  REV : Inport  Port=2
  BRK : Inport  Port=3
  Controlled PWM Voltage : ee_lib/Integrated Circuits/Controlled PWM Voltage  F=400 Hz  TD=0 s  pulse_width_offset=0 s  pulse_min=0 s  pwm_or_av=2  event_type=1  sample_time=1e-6 s  Vmin=0 V  Vmax=5 V  Vm=5 V  u_min=0  u_max=1
  Electrical Reference1 : fl_lib/Electrical/Electrical Elements/Electrical Reference
  H-Bridge : ee_lib/Semiconductors & Converters/Converters/H-Bridge  supply_ports=ee.enum.supply_ports.hidesupply  pwm_or_av=2  regenerative_braking_mode=2  discontinuous=0  freewheeling_mode=1  Rload=10 Ohm  Lload=1e-5 H  F=10 kHz  Venable=2.5 V  Vmax=5 V  Vreverse=2.5 V  Vbrake=2.5 V  Vm=12 V  Ron=0.1 Ohm  Don=0.05 Ohm  Goff=1e-6 S  Tmeas=298.15 K  Ron2=0.1 Ohm  Don2=0.05 Ohm  Tmeas2=398.15 K  thermal_mass=100 J/K  initial_temperature=298.15 K
  SL2Vbrk : Subsystem
  SL2Vduty : Subsystem
  SL2Vrev : Subsystem
  Scope : Scope  NumInputPorts=4
  V + : PMIOPort  Tag=PMCPort  Side=Right
  V -- : PMIOPort  Tag=PMCPort  Port=2  Side=Right
  wires:
  Duty/1 -> Scope/3, SL2Vduty/1(Signal)
  REV/1 -> Scope/2, SL2Vrev/1(Signal)
  BRK/1 -> Scope/4, SL2Vbrk/1(Signal)
  connections:
  Controlled PWM Voltage/RConn2 -- H-Bridge/RConn2 -- V --/RConn1 -- Electrical Reference1/LConn1 -- Controlled PWM Voltage/LConn2 -- H-Bridge/LConn2
  SL2Vrev/RConn1 -- H-Bridge/LConn3
  H-Bridge/RConn1 -- V +/RConn1
  SL2Vduty/RConn1 -- Controlled PWM Voltage/LConn1
  H-Bridge/LConn1 -- Controlled PWM Voltage/RConn1
  SL2Vbrk/RConn1 -- H-Bridge/LConn4

== system cst_robotarm/6 DOF Robot Arm/DC Motors/Wrist Motor/Power Amplifier ==
  Duty : Inport
  REV : Inport  Port=2
  BRK : Inport  Port=3
  Controlled PWM Voltage : ee_lib/Integrated Circuits/Controlled PWM Voltage  F=400 Hz  TD=0 s  pulse_width_offset=0 s  pulse_min=0 s  pwm_or_av=2  event_type=1  sample_time=1e-6 s  Vmin=0 V  Vmax=5 V  Vm=5 V  u_min=0  u_max=1
  Electrical Reference1 : fl_lib/Electrical/Electrical Elements/Electrical Reference
  H-Bridge : ee_lib/Semiconductors & Converters/Converters/H-Bridge  supply_ports=ee.enum.supply_ports.hidesupply  pwm_or_av=2  regenerative_braking_mode=2  discontinuous=0  freewheeling_mode=1  Rload=10 Ohm  Lload=1e-5 H  F=10 kHz  Venable=2.5 V  Vmax=5 V  Vreverse=2.5 V  Vbrake=2.5 V  Vm=12 V  Ron=0.1 Ohm  Don=0.05 Ohm  Goff=1e-6 S  Tmeas=298.15 K  Ron2=0.1 Ohm  Don2=0.05 Ohm  Tmeas2=398.15 K  thermal_mass=100 J/K  initial_temperature=298.15 K
  SL2Vbrk : Subsystem
  SL2Vduty : Subsystem
  SL2Vrev : Subsystem
  V + : PMIOPort  Tag=PMCPort  Side=Right
  V -- : PMIOPort  Tag=PMCPort  Port=2  Side=Right
  wires:
  BRK/1 -> SL2Vbrk/1(Signal)
  REV/1 -> SL2Vrev/1(Signal)
  Duty/1 -> SL2Vduty/1(Signal)
  connections:
  SL2Vbrk/RConn1 -- H-Bridge/LConn4
  H-Bridge/LConn1 -- Controlled PWM Voltage/RConn1
  SL2Vduty/RConn1 -- Controlled PWM Voltage/LConn1
  H-Bridge/RConn1 -- V +/RConn1
  SL2Vrev/RConn1 -- H-Bridge/LConn3
  H-Bridge/LConn2 -- Controlled PWM Voltage/LConn2 -- Electrical Reference1/LConn1 -- V --/RConn1 -- H-Bridge/RConn2 -- Controlled PWM Voltage/RConn2

== system cst_robotarm/6 DOF Robot Arm/6 DOF Robot Arm Mechanics/Forearm/ServoTJD_1_RIGID/ServoHornPlastic_1_RIGID ==
  ReferenceFrame : sm_lib/Frames and Transforms/Reference Frame
  Solid : sm_lib/Body Elements/File Solid  ExtGeomFileName=ServoHornPlastic_Default_sldprt.STL  UnitType=Custom  ExtGeomFileUnits=mm  StepReaderType=HEX  ExportConvexHullGeometry=off  InertiaType=Custom  Mass=0.0010704340009196711  MassUnits=kg  CenterOfMass=[0 -1.2011682426591921 0]  CenterOfMassUnits=mm  MomentsOfInertia=[0.037722424473240444 0.072621190507680802 0.036596357544803754]  MomentsOfInertiaUnits=kg*mm^2  ProductsOfInertia=[0 0 0]  ProductsOfInertiaUnits=kg*mm^2  BasedOnType=Density  Density=1000  DensityUnits=kg/(m^3)  DoExposeReferenceFrame=on  SerializedFrames=<Frames/>  GraphicType=FromGeometry  MarkerShape=Sphere  MarkerSize=10  MarkerSizeUnits=m  GraphicVisPropType=SimpleVisualProperties  GraphicDiffuseColor=[1.0 1.0 1.0]  GraphicSpecularColor=[0.5 0.5 0.5 1.0]  GraphicAmbientColor=[0.15 0.15 0.15 1.0]  GraphicEmissiveColor=[0.0 0.0 0.0 1.0]  GraphicShininess=75  GraphicOpacity=1
  F : PMIOPort  Side=Left
  connections:
  Solid/RConn1 -- ReferenceFrame/RConn1 -- F/RConn1

== system cst_robotarm/6 DOF Robot Arm/6 DOF Robot Arm Mechanics/Forearm/ServoTJD_1_RIGID/bottom_cover_1_RIGID ==
  ReferenceFrame : sm_lib/Frames and Transforms/Reference Frame
  Solid : sm_lib/Body Elements/File Solid  ExtGeomFileName=bottomCover_Default_sldprt.STL  UnitType=Custom  ExtGeomFileUnits=mm  StepReaderType=HEX  ExportConvexHullGeometry=off  InertiaType=Custom  Mass=0.0069725116500885713  MassUnits=kg  CenterOfMass=[0 0.85958385692466177 0]  CenterOfMassUnits=mm  MomentsOfInertia=[0.21879995145338263 1.0303249150901777 0.81533794134290127]  MomentsOfInertiaUnits=kg*mm^2  ProductsOfInertia=[0 0 0]  ProductsOfInertiaUnits=kg*mm^2  BasedOnType=Density  Density=1000  DensityUnits=kg/(m^3)  DoExposeReferenceFrame=on  SerializedFrames=<Frames/>  GraphicType=FromGeometry  MarkerShape=Sphere  MarkerSize=10  MarkerSizeUnits=m  GraphicVisPropType=SimpleVisualProperties  GraphicDiffuseColor=[0.4 0.4 0.4]  GraphicSpecularColor=[0.5 0.5 0.5 1.0]  GraphicAmbientColor=[0.15 0.15 0.15 1.0]  GraphicEmissiveColor=[0.0 0.0 0.0 1.0]  GraphicShininess=75  GraphicOpacity=1
  F : PMIOPort  Side=Left
  connections:
  Solid/RConn1 -- ReferenceFrame/RConn1 -- F/RConn1

== system cst_robotarm/6 DOF Robot Arm/6 DOF Robot Arm Mechanics/Forearm/ServoTJD_1_RIGID/servo_Case_1_RIGID ==
  ReferenceFrame : sm_lib/Frames and Transforms/Reference Frame
  Solid : sm_lib/Body Elements/File Solid  ExtGeomFileName=servoCase_Default_sldprt.STL  UnitType=Custom  ExtGeomFileUnits=mm  StepReaderType=HEX  ExportConvexHullGeometry=off  InertiaType=Custom  Mass=0.024788567791665928  MassUnits=kg  CenterOfMass=[0.08042125391634411 -6.0857711413150408 -0.045303315504018803]  CenterOfMassUnits=mm  MomentsOfInertia=[2.4475554038950817 5.416405903149534 5.3480430794560796]  MomentsOfInertiaUnits=kg*mm^2  ProductsOfInertia=[0.0035757453477574665 0.0080258931443943603 -0.048088274914116991]  ProductsOfInertiaUnits=kg*mm^2  BasedOnType=Density  Density=1000  DensityUnits=kg/(m^3)  DoExposeReferenceFrame=on  SerializedFrames=<Frames/>  GraphicType=FromGeometry  MarkerShape=Sphere  MarkerSize=10  MarkerSizeUnits=m  GraphicVisPropType=SimpleVisualProperties  GraphicDiffuseColor=[0.4 0.4 0.4]  GraphicSpecularColor=[0.5 0.5 0.5 1.0]  GraphicAmbientColor=[0.15 0.15 0.15 1.0]  GraphicEmissiveColor=[0.0 0.0 0.0 1.0]  GraphicShininess=75  GraphicOpacity=1
  F : PMIOPort  Side=Left
  connections:
  Solid/RConn1 -- ReferenceFrame/RConn1 -- F/RConn1

== system cst_robotarm/6 DOF Robot Arm/6 DOF Robot Arm Mechanics/Forearm/ServoTJD_1_RIGID/servo_cover_2_RIGID ==
  ReferenceFrame : sm_lib/Frames and Transforms/Reference Frame
  Solid : sm_lib/Body Elements/File Solid  ExtGeomFileName=servoCover_Default_sldprt.STL  UnitType=Custom  ExtGeomFileUnits=mm  StepReaderType=HEX  ExportConvexHullGeometry=off  InertiaType=Custom  Mass=0.018198073455255783  MassUnits=kg  CenterOfMass=[19.173079671185903 9.8425000000000011 6.6069555093490839]  CenterOfMassUnits=mm  MomentsOfInertia=[1.0514460019053871 4.1870037592553642 4.7863110501402781]  MomentsOfInertiaUnits=kg*mm^2  ProductsOfInertia=[0 0.046415809435786888 0]  ProductsOfInertiaUnits=kg*mm^2  BasedOnType=Density  Density=1000  DensityUnits=kg/(m^3)  DoExposeReferenceFrame=on  SerializedFrames=<Frames/>  GraphicType=FromGeometry  MarkerShape=Sphere  MarkerSize=10  MarkerSizeUnits=m  GraphicVisPropType=SimpleVisualProperties  GraphicDiffuseColor=[0.6 0.6 0.6]  GraphicSpecularColor=[0.5 0.5 0.5 1.0]  GraphicAmbientColor=[0.15 0.15 0.15 1.0]  GraphicEmissiveColor=[0.0 0.0 0.0 1.0]  GraphicShininess=75  GraphicOpacity=1
  F : PMIOPort  Side=Left
  connections:
  Solid/RConn1 -- ReferenceFrame/RConn1 -- F/RConn1

== system cst_robotarm/6 DOF Robot Arm/6 DOF Robot Arm Mechanics/Forearm/ServoTJD_2_RIGID/ServoHornPlastic_1_RIGID ==
  ReferenceFrame : sm_lib/Frames and Transforms/Reference Frame
  Solid : sm_lib/Body Elements/File Solid  ExtGeomFileName=ServoHornPlastic_Default_sldprt.STL  UnitType=Custom  ExtGeomFileUnits=mm  StepReaderType=HEX  ExportConvexHullGeometry=off  InertiaType=Custom  Mass=0.0010704340009196711  MassUnits=kg  CenterOfMass=[0 -1.2011682426591921 0]  CenterOfMassUnits=mm  MomentsOfInertia=[0.037722424473240444 0.072621190507680802 0.036596357544803754]  MomentsOfInertiaUnits=kg*mm^2  ProductsOfInertia=[0 0 0]  ProductsOfInertiaUnits=kg*mm^2  BasedOnType=Density  Density=1000  DensityUnits=kg/(m^3)  DoExposeReferenceFrame=on  SerializedFrames=<Frames/>  GraphicType=FromGeometry  MarkerShape=Sphere  MarkerSize=10  MarkerSizeUnits=m  GraphicVisPropType=SimpleVisualProperties  GraphicDiffuseColor=[1.0 1.0 1.0]  GraphicSpecularColor=[0.5 0.5 0.5 1.0]  GraphicAmbientColor=[0.15 0.15 0.15 1.0]  GraphicEmissiveColor=[0.0 0.0 0.0 1.0]  GraphicShininess=75  GraphicOpacity=1
  F : PMIOPort  Side=Left
  connections:
  Solid/RConn1 -- ReferenceFrame/RConn1 -- F/RConn1

== system cst_robotarm/6 DOF Robot Arm/6 DOF Robot Arm Mechanics/Forearm/ServoTJD_2_RIGID/bottom_cover_1_RIGID ==
  ReferenceFrame : sm_lib/Frames and Transforms/Reference Frame
  Solid : sm_lib/Body Elements/File Solid  ExtGeomFileName=bottomCover_Default_sldprt.STL  UnitType=Custom  ExtGeomFileUnits=mm  StepReaderType=HEX  ExportConvexHullGeometry=off  InertiaType=Custom  Mass=0.0069725116500885713  MassUnits=kg  CenterOfMass=[0 0.85958385692466177 0]  CenterOfMassUnits=mm  MomentsOfInertia=[0.21879995145338263 1.0303249150901777 0.81533794134290127]  MomentsOfInertiaUnits=kg*mm^2  ProductsOfInertia=[0 0 0]  ProductsOfInertiaUnits=kg*mm^2  BasedOnType=Density  Density=1000  DensityUnits=kg/(m^3)  DoExposeReferenceFrame=on  SerializedFrames=<Frames/>  GraphicType=FromGeometry  MarkerShape=Sphere  MarkerSize=10  MarkerSizeUnits=m  GraphicVisPropType=SimpleVisualProperties  GraphicDiffuseColor=[0.4 0.4 0.4]  GraphicSpecularColor=[0.5 0.5 0.5 1.0]  GraphicAmbientColor=[0.15 0.15 0.15 1.0]  GraphicEmissiveColor=[0.0 0.0 0.0 1.0]  GraphicShininess=75  GraphicOpacity=1
  F : PMIOPort  Side=Left
  connections:
  Solid/RConn1 -- ReferenceFrame/RConn1 -- F/RConn1

== system cst_robotarm/6 DOF Robot Arm/6 DOF Robot Arm Mechanics/Forearm/ServoTJD_2_RIGID/servo_Case_1_RIGID ==
  ReferenceFrame : sm_lib/Frames and Transforms/Reference Frame
  Solid : sm_lib/Body Elements/File Solid  ExtGeomFileName=servoCase_Default_sldprt.STL  UnitType=Custom  ExtGeomFileUnits=mm  StepReaderType=HEX  ExportConvexHullGeometry=off  InertiaType=Custom  Mass=0.024788567791665928  MassUnits=kg  CenterOfMass=[0.08042125391634411 -6.0857711413150408 -0.045303315504018803]  CenterOfMassUnits=mm  MomentsOfInertia=[2.4475554038950817 5.416405903149534 5.3480430794560796]  MomentsOfInertiaUnits=kg*mm^2  ProductsOfInertia=[0.0035757453477574665 0.0080258931443943603 -0.048088274914116991]  ProductsOfInertiaUnits=kg*mm^2  BasedOnType=Density  Density=1000  DensityUnits=kg/(m^3)  DoExposeReferenceFrame=on  SerializedFrames=<Frames/>  GraphicType=FromGeometry  MarkerShape=Sphere  MarkerSize=10  MarkerSizeUnits=m  GraphicVisPropType=SimpleVisualProperties  GraphicDiffuseColor=[0.4 0.4 0.4]  GraphicSpecularColor=[0.5 0.5 0.5 1.0]  GraphicAmbientColor=[0.15 0.15 0.15 1.0]  GraphicEmissiveColor=[0.0 0.0 0.0 1.0]  GraphicShininess=75  GraphicOpacity=1
  F : PMIOPort  Side=Left
  connections:
  Solid/RConn1 -- ReferenceFrame/RConn1 -- F/RConn1

== system cst_robotarm/6 DOF Robot Arm/6 DOF Robot Arm Mechanics/Forearm/ServoTJD_2_RIGID/servo_cover_2_RIGID ==
  ReferenceFrame : sm_lib/Frames and Transforms/Reference Frame
  Solid : sm_lib/Body Elements/File Solid  ExtGeomFileName=servoCover_Default_sldprt.STL  UnitType=Custom  ExtGeomFileUnits=mm  StepReaderType=HEX  ExportConvexHullGeometry=off  InertiaType=Custom  Mass=0.018198073455255783  MassUnits=kg  CenterOfMass=[19.173079671185903 9.8425000000000011 6.6069555093490839]  CenterOfMassUnits=mm  MomentsOfInertia=[1.0514460019053871 4.1870037592553642 4.7863110501402781]  MomentsOfInertiaUnits=kg*mm^2  ProductsOfInertia=[0 0.046415809435786888 0]  ProductsOfInertiaUnits=kg*mm^2  BasedOnType=Density  Density=1000  DensityUnits=kg/(m^3)  DoExposeReferenceFrame=on  SerializedFrames=<Frames/>  GraphicType=FromGeometry  MarkerShape=Sphere  MarkerSize=10  MarkerSizeUnits=m  GraphicVisPropType=SimpleVisualProperties  GraphicDiffuseColor=[0.6 0.6 0.6]  GraphicSpecularColor=[0.5 0.5 0.5 1.0]  GraphicAmbientColor=[0.15 0.15 0.15 1.0]  GraphicEmissiveColor=[0.0 0.0 0.0 1.0]  GraphicShininess=75  GraphicOpacity=1
  F : PMIOPort  Side=Left
  connections:
  Solid/RConn1 -- ReferenceFrame/RConn1 -- F/RConn1
